simulink model "psbarcmodels"  (Simulink 6.0)
settings: Solver=ode23tb  StartTime=0.0  StopTime=.04  RelTol=1e-5  AbsTol=1.e-5
libraries: powerlib2 x30
settings Model: Creator=dkennedy  LastModifiedBy=batserve  ExtModeTrigMode=oneshot  ExtModeArmWhenConnect=off  ExtModeAutoUpdateStatusClock=off
settings DataIOCC: LimitDataPoints=off  SignalLoggingName=sigsOut
settings OptimizationCC: BlockReduction=off  BooleanDataType=off
settings DebuggingCC: AlgebraicLoopMsg=none  SolverPrmCheckMsg=none
settings HardwareCC: TargetUnknown=on

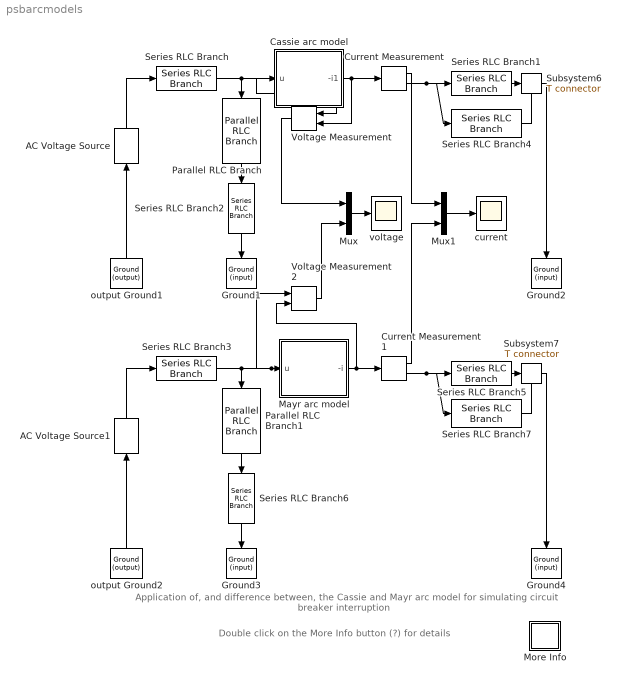
== system psbarcmodels ==
  note: Application of, and difference between, the Cassie and Mayr arc model
      | for simulating circuit breaker interruption
  note: Double click on the More Info button (?) for details
  AC Voltage Source : powerlib2/Electrical Sources/AC Voltage Source  Tag=PoWeRsYsTeMbLoCk  Orientation=up  A=59196  P=90  F=60  stime=0  mesure=None  PSBOutputType=1
  AC Voltage Source1 : powerlib2/Electrical Sources/AC Voltage Source  Tag=PoWeRsYsTeMbLoCk  Orientation=up  A=59196  P=90  F=60  stime=0  mesure=None  PSBOutputType=1
  Cassie arc model : Subsystem  AncestorBlock=arc_model/Cassie arc model  mask(Cassie arc model){tau=1.2e-6, Uc=3850, x0=1.e4, cb_trip=.02}
      mask prompts: tau "tau [s]"; Uc "Uc [V]"; x0 "g(0) [S]"; cb_trip "circuit breaker contact separation starts at [s]"
      mask help: The Cassie arc model with a constant time parameter tau and a constant arc voltage Uc: dlng/dt=1/tau*((u^2/Uc^2)-1.
      mask Help:
      | The Cassie arc model with a constant time parameter tau and a constant arc voltage Uc: dlng/dt=1/tau*((u^2/Uc^2)-1.
      | 
      | The initial conductance of the arc g(0) can be altered. Furthermore, the time at which the contact separation of the circuit breaker takes place can be specified. Until that time the arc model behaves as a conductance with the value g(0).
      mask Display: plot(-15,10,115,90,[-15,15],[50,50],[85,115],[50,50],[15,15,25,25,15],[55,45,45,55,55],[75,75,85,85,75],[55,45,45,55,55],[25,75],[50,70])
  Current Measurement : powerlib2/Measurements/Current Measurement  Tag=PoWeRsYsTeMmEaSuReMeNt  PhasorSimulation=off  OutputType=Magnitude  PSBOutputType=01  PSBequivalent=0
  Current Measurement1 : powerlib2/Measurements/Current Measurement  Tag=PoWeRsYsTeMmEaSuReMeNt  PhasorSimulation=off  OutputType=Magnitude  PSBOutputType=01  PSBequivalent=0
  Ground{1..4} (4 alike) : powerlib2/Connectors/Ground (input)  Tag=PoWeRsYsTeMbLoCk  Orientation=down
  Mayr arc model : Subsystem  AncestorBlock=arc_model/Mayr arc model  mask(Mayr arc model){tau=0.3e-6, P=30900, x0=1.e4, cb_trip=.02}
      mask prompts: tau "tau [s]"; P "P [W]"; x0 "g(0) [S]"; cb_trip "circuit breaker contact separation starts at [s]"
      mask help: The Mayr arc model with a constant time parameter tau and constant cooling power P: dlng/dt=1/tau*((ui/P)-1).
      mask Help:
      | The Mayr arc model with a constant time parameter tau and constant cooling power P: dlng/dt=1/tau*((ui/P)-1).
      | 
      | The initial conductance of the arc g(0) can be altered. Furthermore, the time at which the contact separation of the circuit breaker takes place can be specified. Until that time the arc model behaves as a conductance with the value g(0).
      mask Display: plot(-15,10,115,90,[-15,15],[50,50],[85,115],[50,50],[15,15,25,25,15],[55,45,45,55,55],[75,75,85,85,75],[55,45,45,55,55],[25,75],[50,70])
  More Info : Subsystem
      mask Display: disp('?')
  Mux : Mux  Inputs=2
  Mux1 : Mux  Inputs=2
  Parallel RLC Branch : powerlib2/Elements/Parallel RLC Branch  Tag=PoWeRsYsTeMbLoCk  Orientation=down  a=29.8  b=5.28e-3  c=0  mesure=None  PSBOutputType=1
  Parallel RLC Branch1 : powerlib2/Elements/Parallel RLC Branch  Tag=PoWeRsYsTeMbLoCk  Orientation=down  a=29.8  b=5.28e-3  c=0  mesure=None  PSBOutputType=1
  Series RLC Branch : powerlib2/Elements/Series RLC Branch  Tag=PoWeRsYsTeMbLoCk  a=0  b=3.52e-03  c=inf  mesure=None  PSBOutputType=1
  Series RLC Branch1 : powerlib2/Elements/Series RLC Branch  Tag=PoWeRsYsTeMbLoCk  a=0  b=6.256e-4  c=inf  mesure=None  PSBOutputType=1
  Series RLC Branch2 : powerlib2/Elements/Series RLC Branch  Tag=PoWeRsYsTeMbLoCk  Orientation=down  a=0  b=0  c=1.98e-6  mesure=None  PSBOutputType=1
  Series RLC Branch3 : powerlib2/Elements/Series RLC Branch  Tag=PoWeRsYsTeMbLoCk  a=0  b=3.52e-03  c=inf  mesure=None  PSBOutputType=1
  Series RLC Branch4 : powerlib2/Elements/Series RLC Branch  Tag=PoWeRsYsTeMbLoCk  a=450  b=0  c=1.93e-9  mesure=None  PSBOutputType=1
  Series RLC Branch5 : powerlib2/Elements/Series RLC Branch  Tag=PoWeRsYsTeMbLoCk  a=0  b=6.256e-4  c=inf  mesure=None  PSBOutputType=1
  Series RLC Branch6 : powerlib2/Elements/Series RLC Branch  Tag=PoWeRsYsTeMbLoCk  Orientation=down  a=0  b=0  c=1.98e-6  mesure=None  PSBOutputType=1
  Series RLC Branch7 : powerlib2/Elements/Series RLC Branch  Tag=PoWeRsYsTeMbLoCk  a=450  b=0  c=1.93e-9  mesure=None  PSBOutputType=1
  Subsystem6 : powerlib2/Connectors/T connector  Tag=PoWeRsYsTeMbLoCk  PSBOutputType=1
  Subsystem7 : powerlib2/Connectors/T connector  Tag=PoWeRsYsTeMbLoCk  PSBOutputType=1
  Voltage Measurement : powerlib2/Measurements/Voltage Measurement  Tag=PoWeRsYsTeMmEaSuReMeNt  Orientation=left  PhasorSimulation=off  OutputType=Magnitude  PSBOutputType=0  PSBequivalent=0
  Voltage Measurement2 : powerlib2/Measurements/Voltage Measurement  Tag=PoWeRsYsTeMmEaSuReMeNt  PhasorSimulation=off  OutputType=Magnitude  PSBOutputType=0  PSBequivalent=0
  current : Scope
      settings: TimeRange=0.04  YMin=-40000  YMax=40000
  output Ground1 : powerlib2/Connectors/Ground (output)  Tag=PoWeRsYsTeMbLoCk  Orientation=up  PSBOutputType=1
  output Ground2 : powerlib2/Connectors/Ground (output)  Tag=PoWeRsYsTeMbLoCk  Orientation=up  PSBOutputType=1
  voltage : Scope
      settings: TimeRange=0.04  YMin=-100000  YMax=60000
  wires:
  output Ground1/1 -> AC Voltage Source/1
  Parallel RLC Branch/1 -> Series RLC Branch2/1
  Series RLC Branch2/1 -> Ground1/1
  AC Voltage Source/1 -> Series RLC Branch/1
  Series RLC Branch/1 -> Parallel RLC Branch/1, Cassie arc model/1(u), Voltage Measurement/1
  Voltage Measurement/1 -> Mux/1
  Voltage Measurement2/1 -> Mux/2
  Subsystem6/1 -> Ground2/1
  Current Measurement/2 -> Series RLC Branch1/1, Series RLC Branch4/1
  Series RLC Branch1/1 -> Subsystem6/1
  Series RLC Branch4/1 -> Subsystem6/Enable
  Cassie arc model/1(-i1) -> Voltage Measurement/2, Current Measurement/1
  output Ground2/1 -> AC Voltage Source1/1
  Parallel RLC Branch1/1 -> Series RLC Branch6/1
  Series RLC Branch6/1 -> Ground3/1
  AC Voltage Source1/1 -> Series RLC Branch3/1
  Series RLC Branch3/1 -> Parallel RLC Branch1/1, Mayr arc model/1(u), Voltage Measurement2/1
  Subsystem7/1 -> Ground4/1
  Current Measurement1/2 -> Series RLC Branch5/1, Series RLC Branch7/1
  Series RLC Branch5/1 -> Subsystem7/1
  Series RLC Branch7/1 -> Subsystem7/Enable
  Mayr arc model/1(-i) -> Voltage Measurement2/2, Current Measurement1/1
  Mux/1 -> voltage/1
  Mux1/1 -> current/1
  Current Measurement/1 -> Mux1/1
  Current Measurement1/1 -> Mux1/2

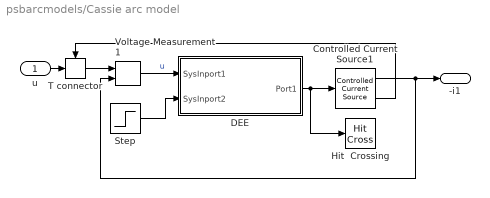
== system psbarcmodels/Cassie arc model ==
  u : Inport  Port=1  LatchInput=off
  Controlled Current Source1 : powerlib2/Electrical Sources/Controlled Current Source  Tag=PoWeRsYsTeMbLoCk  initsrc=on  srctyp=AC  ia=0  iph=0  freq=0  mesure=None  PSBOutputType=11
  DEE : Subsystem
      settings: OpenFcn=diffeqed
      mask Type: Differential Equation Editor (DEE)
      mask Display: disp('Cassie arc model')
  Hit  Crossing : HitCross  ZeroCross=off  ShowOutputPort=off
  Step : Step  Time=cb_trip  SampleTime=0  ZeroCross=off
  T connector : powerlib2/Connectors/T connector  Tag=PoWeRsYsTeMbLoCk  PSBOutputType=1
  Voltage Measurement1 : powerlib2/Measurements/Voltage Measurement  Tag=PoWeRsYsTeMmEaSuReMeNt  PhasorSimulation=off  OutputType=Magnitude  PSBOutputType=0  PSBequivalent=0
  -i1 : Outport
  wires:
  Step/1 -> DEE/2(SysInport2)
  DEE/1(Port1) -> Hit  Crossing/1, Controlled Current Source1/1
  Controlled Current Source1/1 -> -i1/1, Voltage Measurement1/2
  Controlled Current Source1/2 -> T connector/Enable
  T connector/1 -> Voltage Measurement1/1
  u/1 -> T connector/1
  Voltage Measurement1/1 -> DEE/1(SysInport1)  "u"

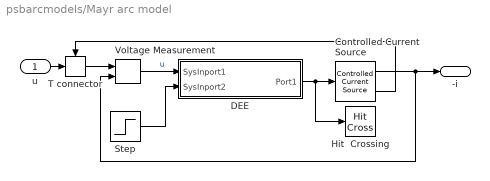
== system psbarcmodels/Mayr arc model ==
  u : Inport  Port=1  LatchInput=off
  Controlled Current Source : powerlib2/Electrical Sources/Controlled Current Source  Tag=PoWeRsYsTeMbLoCk  initsrc=on  srctyp=AC  ia=0  iph=0  freq=0  mesure=None  PSBOutputType=11
  DEE : Subsystem
      settings: OpenFcn=diffeqed
      mask Type: Differential Equation Editor (DEE)
      mask Display: disp('Mayr arc model')
  Hit  Crossing : HitCross  ZeroCross=off  ShowOutputPort=off
  Step : Step  Time=cb_trip  SampleTime=0  ZeroCross=off
  T connector : powerlib2/Connectors/T connector  Tag=PoWeRsYsTeMbLoCk  PSBOutputType=1
  Voltage Measurement : powerlib2/Measurements/Voltage Measurement  Tag=PoWeRsYsTeMmEaSuReMeNt  PhasorSimulation=off  OutputType=Magnitude  PSBOutputType=0  PSBequivalent=0
  -i : Outport
  wires:
  Step/1 -> DEE/2(SysInport2)
  DEE/1(Port1) -> Hit  Crossing/1, Controlled Current Source/1
  Controlled Current Source/1 -> Voltage Measurement/2, -i/1
  Controlled Current Source/2 -> T connector/Enable
  T connector/1 -> Voltage Measurement/1
  u/1 -> T connector/1
  Voltage Measurement/1 -> DEE/1(SysInport1)  "u"

== system psbarcmodels/More Info ==
  note: Two identical circuits are displayed: one with a Cassie and one with a Mayr arc model.
      | The circuit is a simple representation of a circuit breaker interrupting a short-line fault.
      | At the source side of the circuit breaker a circuit is present for reproducing a (2-parameter
      | IEC) transient recovery voltage, while the RLC circuit at the line side represents a short
      | transmission line that is short circuited.
      |
      | A stiff solver is recommended for this type of problems due to the nonlinear
      | behaviour of the arc.
  note: This demonstration illustrates use of the Cassie and Mayr arc model
      | for simulating high voltage circuit breaker interruption
  note: Demonstration
  note: Circuit Description
  note: A blockset containing 7 arc models can be downloaded freely from the following website of the
      | Power Systems Laboratory of the Delft University of Technology: eps.et.tudelft.nl
      | A PDF manual with installation instructions, arc model descriptions and references to relevant
      | literature is included.
  note: Arc Model Blockset: eps.et.tudelft.nl
  note: The circuit breaker interruption can be started by means of the 'Start/Pause Simulation' button.
      | The voltages over both the Cassie (yellow) and Mayr arc model are displayed in one scope.
      | The currents through both the Cassie (yellow) and Mayr arc model are displayed in one scope.
      |
      | The following observations become clear from the simulation:
      | The arc behaves as a non-linear resistance; therefore both arc current and voltage pass
      | the zero value at the same time. As the power input into the arc channel is zero
      | at that time, the current zero crossing is the place where the interruption takes
      | place.
      |
      | The Cassie arc model has a constant arc voltage in the high current interval, while the
      | Mayr arc model shows an increasing arc voltage (the extinction peak) close to the
      | current zero crossing.
      |
      | The Cassie arc model fails to interrupt the short circuit current, while the Mayr arc model
      | interrupts and shows a small post-arc current of 0.6A immediately after the current zero
      | crossing. This current is caused by the transient recovery voltage building up over the
      | non-infinite arc resistance.
      |
      | In case of the Mayr arc model (the successfull interruption), the transient recovery voltage
      | (TRV) builds up over the breaker. This voltage consists of the 2-parameter TRV and the high
      | frequency voltage oscillation of the line side, which can be observed by zooming in.
  note: P.H. Schavemaker, Power Systems Laboratory,
      | Delft University of Technology, the Netherlands
      |
      | P.H.Schavemaker@its.tudelft.nl

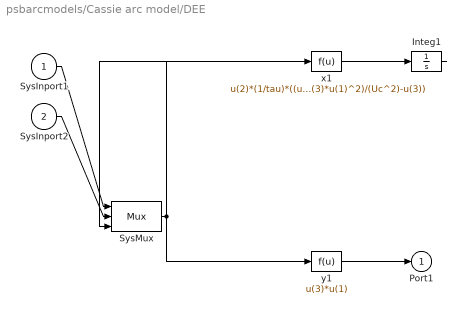
== system psbarcmodels/Cassie arc model/DEE ==
  SysInport1 : Inport  Port=1  LatchInput=off
  SysInport2 : Inport  Port=2  LatchInput=off
  Integ1 : Integrator  InitialCondition=x0  ZeroCross=off
  SysMux : Mux  Inputs=3
  x1 : Fcn  Expr=u(2)*(1/tau)*((u(3)*u(1)^2)/(Uc^2)-u(3))
  y1 : Fcn  Expr=u(3)*u(1)
  Port1 : Outport  InitialOutput=0
  wires:
  SysInport1/1 -> SysMux/1
  SysInport2/1 -> SysMux/2
  SysMux/1 -> x1/1, y1/1
  x1/1 -> Integ1/1
  Integ1/1 -> SysMux/3
  y1/1 -> Port1/1

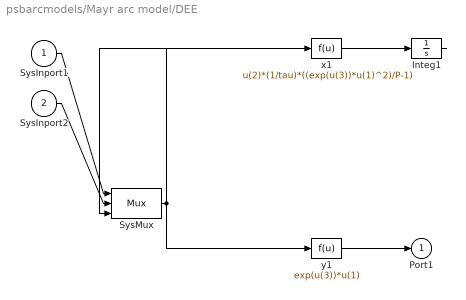
== system psbarcmodels/Mayr arc model/DEE ==
  SysInport1 : Inport  Port=1  LatchInput=off
  SysInport2 : Inport  Port=2  LatchInput=off
  Integ1 : Integrator  InitialCondition=log(x0)  ZeroCross=off
  SysMux : Mux  Inputs=3
  x1 : Fcn  Expr=u(2)*(1/tau)*((exp(u(3))*u(1)^2)/P-1)
  y1 : Fcn  Expr=exp(u(3))*u(1)
  Port1 : Outport  InitialOutput=0
  wires:
  y1/1 -> Port1/1
  SysMux/1 -> y1/1, x1/1
  Integ1/1 -> SysMux/3
  x1/1 -> Integ1/1
  SysInport2/1 -> SysMux/2
  SysInport1/1 -> SysMux/1
